simulink model "Test_Piero"  (R2023b)
settings: Solver=FixedStepAuto  StartTime=0.0  StopTime=inf  RelTol=1e-3  EnableMultiTasking=on
settings Model: SimulationMode=external  ExtModeTrigDuration=2  Creator=m4ttn  LastModifiedBy=m4ttn
settings SolverCC: AutoInsertRateTranBlk=on
settings OptimizationCC: EnhancedBackFolding=on  PassReuseOutputArgsAs=Individual arguments  ZeroExternalMemoryAtStartup=off  ZeroInternalMemoryAtStartup=off  MaxStackSize=64  OptimizeBlockOrder=speed  DifferentSizesBufferReuse=on  OptimizationCustomize=off  EfficientTunableParamExpr=on
settings DebuggingCC: ParameterTunabilityLossMsg=error
settings HardwareCC: ProdBitPerInt=16  ProdBitPerPointer=16  ProdBitPerSizeT=16  ProdBitPerPtrDiffT=16  ProdLargestAtomicFloat=None  ProdWordSize=8  ProdHWDeviceType=Atmel->AVR  UseEmbeddedCoderFeatures=off  UseSimulinkCoderFeatures=off
settings SFSimCC: MATLABDynamicMemAlloc=off
settings RTWCC: Description=Embedded Coder  SystemTargetFile=ert.tlc  HardwareBoard=Arduino Mega 2560  TLCOptions="-aInlineSetEventsForThisBaseRateFcn=TLC_FALSE -aSuppressMultiTaskScheduler=TLC_FALSE   -aRateBasedStepFcn=1"  TemplateMakefile=ert_default_tmf  Toolchain=Arduino AVR  BuildConfiguration=Faster Runs  GPUComputeCapability=5.0
settings CodeAppCC: ForceParamTrailComments=on  IgnoreCustomStorageClasses=off  OperatorAnnotations=on  SimulinkDataObjDesc=on  SFDataObjDesc=on  InsertBlockDesc=on
settings ERTTargetCC: SupportContinuousTime=on  SupportNonInlinedSFcns=on  SupportVariableSizeSignals=on  ExtModeTransport=3  ExtModeStaticAlloc=on  ExtModeAutomaticAllocSize=off  ExtModeStaticAllocSize=2048  ExtModeMexFile=ext_xcp  ExtModeIntrfLevel=Level2 - Open

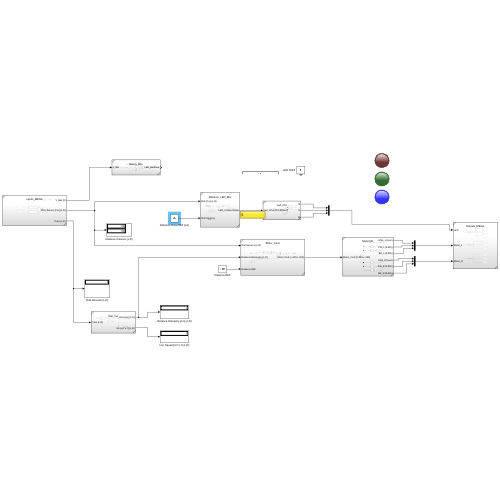
[thumbnail: Simulink's stored preview of the top-level diagram]
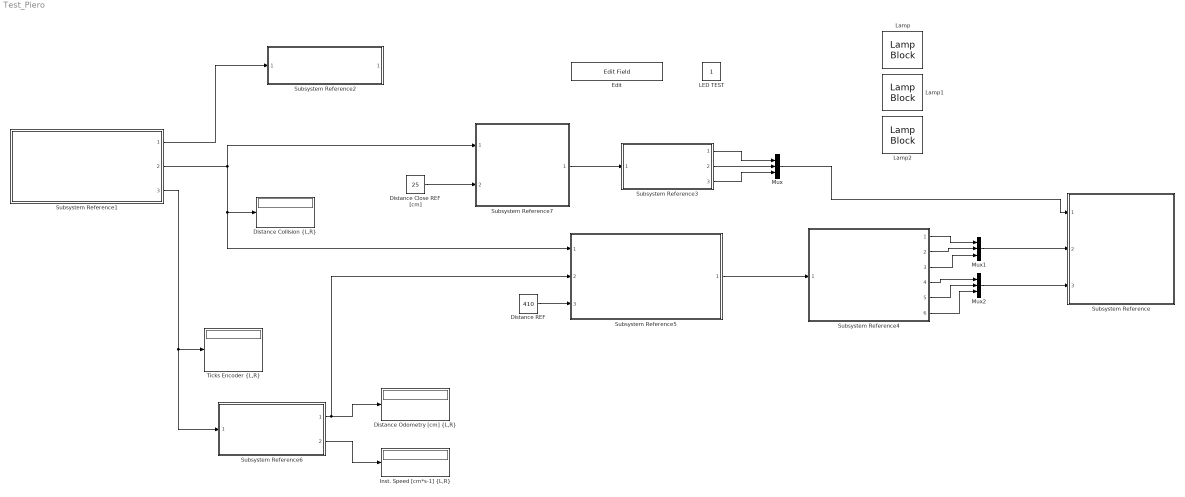
== system Test_Piero ==
  Distance Close REF [cm] : Constant  Value=25  OutDataTypeStr=int16
  "Distance Collision {L,R}" : Display
  "Distance Odometry [cm] {L,R}" : Display
  Distance REF : Constant  Value=410  OutDataTypeStr=int16
  Edit : EditField  LabelPosition=Hide  ShowInitialText=on  Alignment=Center
  "Inst. Speed [cm*s-1] {L,R}" : Display
  LED TEST : Constant  OutDataTypeStr=uint8
  Lamp : LampBlock  LabelPosition=Hide
  Lamp1 : LampBlock  LabelPosition=Hide
  Lamp2 : LampBlock  LabelPosition=Hide
  Mux : Mux  Inputs=3
  Mux1 : Mux  Inputs=3
  Mux2 : Mux  Inputs=3
  Subsystem Reference : Subsystem  ReferencedSubsystem=Outputs_MEGA
  Subsystem Reference1 : Subsystem  ReferencedSubsystem=Inputs_MEGA
  Subsystem Reference2 : Subsystem  ReferencedSubsystem=Batery_Bhv
  Subsystem Reference3 : Subsystem  ReferencedSubsystem=Led_Ctrl
  Subsystem Reference4 : Subsystem  ReferencedSubsystem=MotorCtrl
  Subsystem Reference5 : Subsystem  ReferencedSubsystem=Motor_Cmd
  Subsystem Reference6 : Subsystem  ReferencedSubsystem=Dist_Vel
  Subsystem Reference7 : Subsystem  ReferencedSubsystem=Distance_LED_Bhv
  "Ticks Encoder {L,R}" : Display
  wires:
  Subsystem Reference3/1 -> Mux/1
  Subsystem Reference3/2 -> Mux/2
  Subsystem Reference3/3 -> Mux/3
  Mux/1 -> Subsystem Reference/1
  Subsystem Reference4/1 -> Mux1/1
  Subsystem Reference4/2 -> Mux1/2
  Subsystem Reference4/3 -> Mux1/3
  Subsystem Reference4/4 -> Mux2/1
  Subsystem Reference4/5 -> Mux2/2
  Subsystem Reference4/6 -> Mux2/3
  Mux1/1 -> Subsystem Reference/2
  Mux2/1 -> Subsystem Reference/3
  Subsystem Reference1/1 -> Subsystem Reference2/1
  Subsystem Reference1/2 -> Subsystem Reference7/1, Subsystem Reference5/1, "Distance Collision {L,R}"/1
  Subsystem Reference1/3 -> Subsystem Reference6/1, "Ticks Encoder {L,R}"/1
  Subsystem Reference6/1 -> Subsystem Reference5/2, "Distance Odometry [cm] {L,R}"/1
  Subsystem Reference6/2 -> "Inst. Speed [cm*s-1] {L,R}"/1
  Subsystem Reference7/1 -> Subsystem Reference3/1
  Distance Close REF [cm]/1 -> Subsystem Reference7/2
  Subsystem Reference5/1 -> Subsystem Reference4/1
  Distance REF/1 -> Subsystem Reference5/3
